simulink model "DCMotor_PI_Z_controller_org"  (Simulink 10.0)
settings: Solver=ode45  StartTime=0.0  StopTime=40  FixedStep=0.05  RelTol=1e-3  EnableMultiTasking=on
undefined symbols (not defined in the file): REAL, TIME
libraries: RT x1
settings Model: Creator=Admin  LastModifiedBy=bhisma  ExtModeTrigDuration=5000
settings SolverCC: PositivePriorityOrder=on
settings DataIOCC: LimitDataPoints=on
settings DebuggingCC: StateNameClashWarn=warning
settings RTWCC: Description=QUARC Win64 Target  SystemTargetFile=quarc_win64.tlc  TemplateMakefile=quarc_default_tmf
settings STFCustomTargetCC: TargetPreCompLibLocation=C:\PROGRA~3\QUARC\lib\2013a\win64\release  GeneratePreprocessorConditionals=Disable all  CombineOutputUpdateFcns=on  CPPClassGenCompliant=on  GRTInterface=off  SystemTargetFile=quarc_win64.tlc
settings GRTTargetCC: TargetPreCompLibLocation=C:\PROGRA~3\QUARC\lib\2013a\win64\release  ParMdlRefBuildCompliant=off  CompOptLevelCompliant=off  ConcurrentExecutionCompliant=off  GeneratePreprocessorConditionals=Disable all  CombineOutputUpdateFcns=on  MatFileLogging=off  GRTInterface=off  UseToolchainInfoCompliant=off  ExtMode=on  ExtModeMexFile=quarc_comm
settings ConfigComp: CovExternalEMLEnable=off

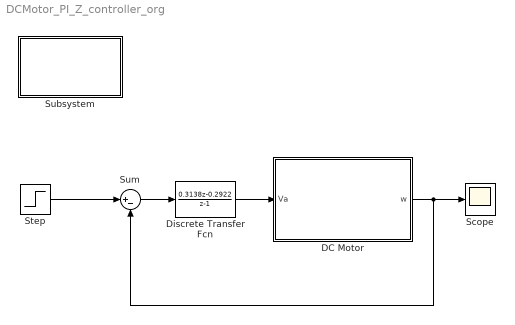
== system DCMotor_PI_Z_controller_org ==
  DC Motor : Subsystem  mask{Ts=0.05}
      mask prompts: Ts "Sample time (Ts)"
      mask Display:
      | image('img/dcmotor.png')
      | port_label('output', 1, 'w')
      | port_label('input', 1, 'Va')
  Discrete Transfer Fcn : DiscreteTransferFcn  Numerator=[0.3138,-0.2922]  Denominator=[1,-1]  SampleTime=0.05
  Scope : Scope
  Step : Step  Time=20  Before=2.5  After=4.5  SampleTime=0.05
  Subsystem : Subsystem
      mask Display: image('img/logo.png')
  Sum : Sum  Inputs=|+-
  wires:
  DC Motor/1(w) -> Sum/2, Scope/1
  Step/1 -> Sum/1
  Sum/1 -> Discrete Transfer Fcn/1
  Discrete Transfer Fcn/1 -> DC Motor/1(Va)

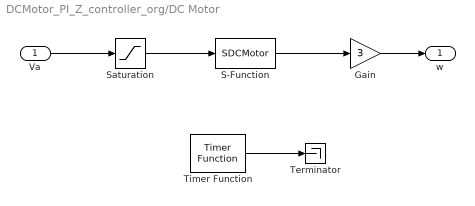
== system DCMotor_PI_Z_controller_org/DC Motor ==
  Va : Inport
  Gain : Gain  Gain=3  SampleTime=Ts
  S-Function : S-Function  FunctionName=SDCMotor  Parameters=Ts  SFunctionDeploymentMode=off  EnableBusSupport=off
  Saturation : Saturate  UpperLimit=10  LowerLimit=0  SampleTime=Ts
  Terminator : Terminator
  Timer Function : RT/Timer Function  Priority=746934680  step=Ts*1000  TaskPriority=REAL-TIME  ThPriority=TIME CRITICAL
  w : Outport
  wires:
  S-Function/1 -> Gain/1
  Va/1 -> Saturation/1
  Saturation/1 -> S-Function/1
  Gain/1 -> w/1
  Timer Function/1 -> Terminator/1

== system DCMotor_PI_Z_controller_org/Subsystem ==
